simulink model "AIE_HDL"  (R2023a)
settings: Solver=FixedStepDiscrete  StartTime=0.0  StopTime=100*2e-9  RelTol=1e-3
InitFcn:
  | xlEvaluateHDLBlocks('AIE_HDL')
undefined symbols (not defined in the file): S, vsva2197, xcvc1902
libraries: hdlUtilities x4, dspsrcs4 x3, aieBasic x3, hdlBasic x2, vmcUtilities x1
settings Model: Creator=shirazi  LastModifiedBy=robg
settings SolverCC: AlgebraicLoopSolver=TrustRegion
settings DebuggingCC: UnconnectedInputMsg=warning  UnconnectedOutputMsg=warning  UnconnectedLineMsg=warning
settings ModelReferenceCC: EnableRefExpFcnMdlSchedulingChecks=on
settings SFSimCC: CustomCodeUndefinedFunction=UseInterfaceOnly
settings RTWCC: DLArmComputeVersion=19.05

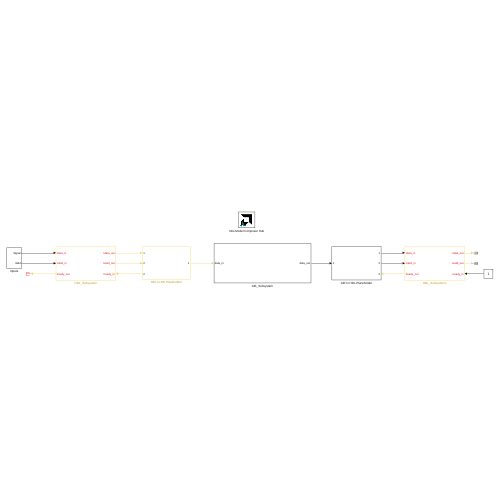
[thumbnail: Simulink's stored preview of the top-level diagram]
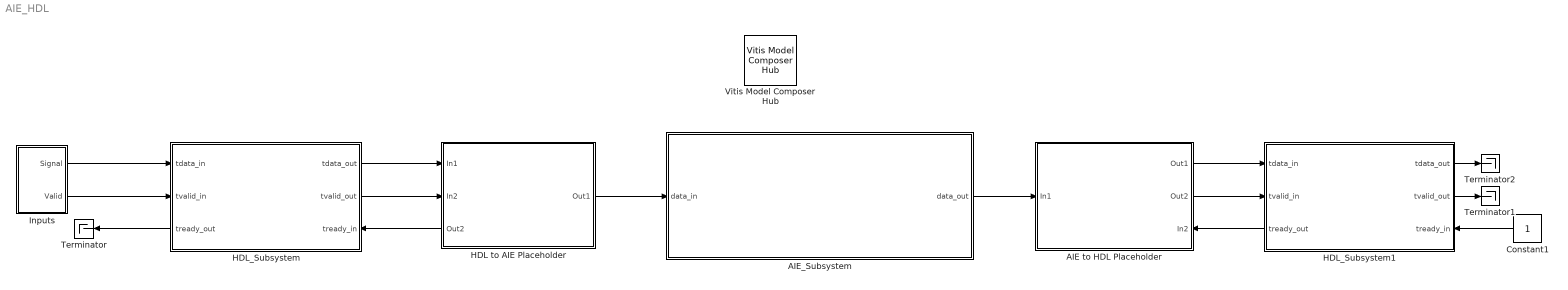
== system AIE_HDL ==
  AIE to HDL Placeholder : Subsystem
      settings: PortSchema="{\"entries\":[{\"content\":{\"sides\":[{\"content\":{\"connectorIds\":[\"In1\"]},\"type\":\"ConnectorPlacement.EquallySpacedRectSide\",\"uuid\":\"7ec462a4-9987-47a7-8ef6-3d77f6cbc297\"},{\"content\":{\"connectorIds\":[\"Out1\",\"Out2\",\"In2\"],\"side\":\"RIGHT\"},\"type\":\"ConnectorPlacement.EquallySpacedRectSide\",\"uuid\":\"048d0a02-5e23-4721-b2a0-067b0b8ade54\"},{\"content\":{\"connectorIds\":[],\"side\":\"TOP\"},\"type\":\"ConnectorPlacement.EquallySpacedRectSide\",\"uuid\":\"3a217202-6b4d-4910-945d-076f614a2b79\"}]},\"type\":\"ConnectorPlacement.EquallySpacedConnector\",\"uuid\":\"7ab6b02b-881c-4c80-a03f-a259c9ab4081\"}],\"packageUris\":[\"http://schema.mathworks.com/mf0/Connector/R2020b\"],\"version\":\"1.0\"}"
  AIE_Subsystem : Subsystem
  Constant1 : Constant  OutDataTypeStr=boolean  SampleTime=2e-9
  HDL to AIE Placeholder : Subsystem
      settings: PortSchema="{\"entries\":[{\"content\":{\"sides\":[{\"content\":{\"connectorIds\":[\"In1\",\"In2\",\"Out2\"]},\"type\":\"ConnectorPlacement.EquallySpacedRectSide\",\"uuid\":\"7ec462a4-9987-47a7-8ef6-3d77f6cbc297\"},{\"content\":{\"connectorIds\":[\"Out1\"],\"side\":\"RIGHT\"},\"type\":\"ConnectorPlacement.EquallySpacedRectSide\",\"uuid\":\"048d0a02-5e23-4721-b2a0-067b0b8ade54\"},{\"content\":{\"connectorIds\":[],\"side\":\"TOP\"},\"type\":\"ConnectorPlacement.EquallySpacedRectSide\",\"uuid\":\"3a217202-6b4d-4910-945d-076f614a2b79\"}]},\"type\":\"ConnectorPlacement.EquallySpacedConnector\",\"uuid\":\"7ab6b02b-881c-4c80-a03f-a259c9ab4081\"}],\"packageUris\":[\"http://schema.mathworks.com/mf0/Connector/R2020b\"],\"version\":\"1.0\"}"
  HDL_Subsystem : Subsystem
      settings: PortSchema="{\"entries\":[{\"content\":{\"sides\":[{\"content\":{\"connectorIds\":[\"In1\",\"In2\",\"Out3\"]},\"type\":\"ConnectorPlacement.EquallySpacedRectSide\",\"uuid\":\"989cb16a-31ef-4a7b-a4d3-adb9fa6297fb\"},{\"content\":{\"connectorIds\":[\"Out1\",\"Out2\",\"In3\"],\"side\":\"RIGHT\"},\"type\":\"ConnectorPlacement.EquallySpacedRectSide\",\"uuid\":\"9f541dfa-b9f2-4468-aad7-758d6944575e\"},{\"content\":{\"connectorIds\":[],\"side\":\"TOP\"},\"type\":\"ConnectorPlacement.EquallySpacedRectSide\",\"uuid\":\"c3c29352-583e-46d2-970b-15c15d07c124\"}]},\"type\":\"ConnectorPlacement.EquallySpacedConnector\",\"uuid\":\"c80158a0-6c2e-4236-83b1-850c61320738\"}],\"packageUris\":[\"http://schema.mathworks.com/mf0/Connector/19700101\"],\"version\":\"1.0\"}"
  HDL_Subsystem1 : Subsystem
      settings: PortSchema="{\"entries\":[{\"content\":{\"sides\":[{\"content\":{\"connectorIds\":[\"In1\",\"In2\",\"Out3\"]},\"type\":\"ConnectorPlacement.EquallySpacedRectSide\",\"uuid\":\"989cb16a-31ef-4a7b-a4d3-adb9fa6297fb\"},{\"content\":{\"connectorIds\":[\"Out1\",\"Out2\",\"In3\"],\"side\":\"RIGHT\"},\"type\":\"ConnectorPlacement.EquallySpacedRectSide\",\"uuid\":\"9f541dfa-b9f2-4468-aad7-758d6944575e\"},{\"content\":{\"connectorIds\":[],\"side\":\"TOP\"},\"type\":\"ConnectorPlacement.EquallySpacedRectSide\",\"uuid\":\"c3c29352-583e-46d2-970b-15c15d07c124\"}]},\"type\":\"ConnectorPlacement.EquallySpacedConnector\",\"uuid\":\"c80158a0-6c2e-4236-83b1-850c61320738\"}],\"packageUris\":[\"http://schema.mathworks.com/mf0/Connector/19700101\"],\"version\":\"1.0\"}"
  Inputs : Subsystem
  Terminator : Terminator
  Terminator1 : Terminator
  Terminator2 : Terminator
  Vitis Model Composer Hub : vmcUtilities/Vitis Model Composer Hub  Tag=genX  CodeGeneration=off  SubsystemName=HDL_Subsystem  StartColumn=1  NumberOfColumns=1  TargetDirectory=./code  exportDesign=off  analyzeDesign=off  validateDesignOnHw=off  ExportType=AI Engines  IpVendor=xilinx.com  IpLibrary=hls  IpVersion=1.0  IpHWLanguage=Verilog  AieCompilerOptions={}  AieSimulatorOptions={}  CreateTestbench=off  TestbenchStackSize=10  RunRtlSim=off  RunCSim=off  RunAieSim=off  AieSimTimeout=50000  RunAieSimProfiling=off  LaunchVitisAnalyzer=off  PlotOutput=off  RunX86Sim=off  X86SimTimeout=10  GenHwImage=off  GenLibadfXo=off  GenHwValidationCode=off  PlatformType=Not Specified  HwSystemType=Baremetal  HwValidationTarget=hw  ProjDevice=xcvc1902-vsva2197-1LP-e-S  ProjDevicePart=xcvc1902-vsva2197-1LP-e-S  AIEType=AIE  SamplePeriod=-1  ClockFrequency=200  DataPathParallelism=1  xilinxfamily=versalaicore  part=xcvc1902  speed=-1LP-e-S  package=vsva2197  directory=./netlist/ip/HDL_Subsystem/src  testbench=off  incr_netlist=off  synthesis_tool=Vivado  clock_wrapper=Clock Enables  dbl_ovrd=According to Block Masks  dcm_input_clock_period=10  sysclk_period=2  simulink_period=2e-9  eval_field=0  LogFileName=''  NThreads=4
  wires:
  HDL to AIE Placeholder/1(Out1) -> AIE_Subsystem/1(data_in)
  HDL_Subsystem/1(tdata_out) -> HDL to AIE Placeholder/1(In1)
  HDL_Subsystem/2(tvalid_out) -> HDL to AIE Placeholder/2(In2)
  HDL to AIE Placeholder/2(Out2) -> HDL_Subsystem/3(tready_in)
  HDL_Subsystem/3(tready_out) -> Terminator/1
  AIE_Subsystem/1(data_out) -> AIE to HDL Placeholder/1(In1)
  AIE to HDL Placeholder/1(Out1) -> HDL_Subsystem1/1(tdata_in)
  AIE to HDL Placeholder/2(Out2) -> HDL_Subsystem1/2(tvalid_in)
  HDL_Subsystem1/3(tready_out) -> AIE to HDL Placeholder/2(In2)
  Constant1/1 -> HDL_Subsystem1/3(tready_in)
  Inputs/1(Signal) -> HDL_Subsystem/1(tdata_in)
  Inputs/2(Valid) -> HDL_Subsystem/2(tvalid_in)
  HDL_Subsystem1/2(tvalid_out) -> Terminator1/1
  HDL_Subsystem1/1(tdata_out) -> Terminator2/1

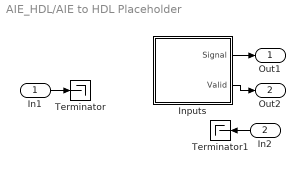
== system AIE_HDL/AIE to HDL Placeholder ==
  In1 : Inport
  In2 : Inport  Port=2
  Inputs : Subsystem
  Terminator : Terminator
  Terminator1 : Terminator
  Out1 : Outport
  Out2 : Outport  Port=2
  wires:
  Inputs/1(Signal) -> Out1/1
  Inputs/2(Valid) -> Out2/1
  In1/1 -> Terminator/1
  In2/1 -> Terminator1/1

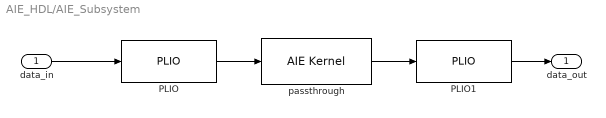
== system AIE_HDL/AIE_Subsystem ==
  data_in : Inport
  PLIO : aieBasic/PLIO  PlioWidth=64  PlioFreqSpec=on  PlioFreq=500  ColLocation=0  channel=0  blockJsonConstraints=[]  deprecateConstraints=0
  PLIO1 : aieBasic/PLIO  PlioWidth=64  PlioFreqSpec=on  PlioFreq=500  ColLocation=0  channel=0  blockJsonConstraints=[]  deprecateConstraints=0
  passthrough : aieBasic/AIE Kernel  KernelAllAttrs=|  PortNames={'in'; 'out'}  PortSerializedTypes={'{R{Tadf::input_buffer{1{t{Bi32}}}}}'; '{R{Tadf::output_buffer{1{t{Bi32}}}}}'}  PortWindowSizes={1.600000000000000000e+01, 1.600000000000000000e+01}  PortWindowMargins={0.000000000000000000e+00, 0.000000000000000000e+00}  PortSynchronicities={'sync', 'sync'}  PortSignalSizes={0.000000000000000000e+00; 0.000000000000000000e+00}  FunctionTemplateSpecKind=implicit  FunctionTemplateParamNames={'FRAME_LENGTH'}  FunctionTemplateParamKinds={'nontype'}  FunctionTemplateParamTypes={'int'}  FunctionTemplateParamValues={'16'}  FunctionIndex=1  FunctionTabVisible=on  FunctionTemplateParamsVisible=on  FunctionDeclTypeOptions=|  FunctionDecl=|  FunctionTemplateParams={ 'FRAME_LENGTH', 'int', '16' }  FunctionTemplateParamsEnables={'off', 'off', 'on'}  PortAttrs={ 'input', 'in', 'adf::input_buffer< int32 > &', '16', '0', 'sync', ''; 'output', 'out', 'adf::output_buffer< int32 > &', '16', '', 'sync', '' }  PortAttrsEnables={'off', 'off', 'off', 'on', 'off', 'off', 'off';'off', 'off', 'off', 'on', 'off', 'off', 'off'}  SampleTime=-1  KernelHeaderFile=passthrough.h  KernelFunction=passthrough  KernelSourceFile=passthrough.cc  KernelSearchPaths={}  PreProcOptions={}  blockJsonConstraints=[]
      KernelAllAttrs=|
      | s[12;12;9;9;19;14;21;23;21;23;24;21;15;17;12;24;26;26;26;27;28;9;21;23;23;23;24;25;14;19;19;29]@FunctionNameDeclFileNamePortNamesPortTypesPortSerializedTypesPortDirectionsPortWindowSizeEnablesPortWindowMarginEnablesPortBufferSizeEnablesPortBufferMarginEnablesPortSynchronicityEnablesPortSignalSizeEnablesPortBufferSizesPortBufferMarginsFunctionDeclFunctionTemplateSpecKindFunctionTemplateParamNamesFunctionTemplateParamKindsFunctionTemplateParamTypesFunctionTemplateParamValuesFunctionTemplateParamEnablesClassDeclClassTemplateSpecKindClassTemplateParamNamesClassTemplateParamKindsClassTemplateParamTypesClassTemplateParamValuesClassTemplateParamEnablesClassCtorDeclsClassCtorParamNamesClassCtorParamTypesClassCtorParamSerializedTypes[1 1]@C[32 1]@t11@passthrought19@../../passthrough.hC[2 1]@t2@int3@outC[2 1]@t28@adf::input_buffer< int32 > &t29@adf::output_buffer< int32 > &C[2 1]@t35@{R{Tadf::input_buffer{1{t{Bi32}}}}}t36@{R{Tadf::output_buffer{1{t{Bi32}}}}}C[2 1]@t5@inputt6@outputC[2 1]@l1@l1@C[2 1]@l1@l0@C[2 1]@l1@l1@C[2 1]@l0@l0@C[2 1]@l1@l1@C[2 1]@l0@l0@C[2 1]@nnC[2 1]@nnt115@template < int FRAME_LENGTH > 
      | void passthrough(adf::input_buffer< int32 > & in, adf::output_buffer< int32 > & out)t8@implicitC[1 1]@t12@FRAME_LENGTHC[1 1]@t7@nontypeC[1 1]@t3@intC[1 1]@nC[1 1]@l1@nne[0 1]@e[0 1]@e[0 1]@e[0 1]@e[0 1]@e[0 1]@e[0 1]@e[0 1]@e[0 1]@
      FunctionDeclTypeOptions=|
      | C[1 1]@t117@template < int FRAME_LENGTH > 
      | void passthrough(adf::input_buffer< int32 > && in, adf::output_buffer< int32 > && out)
      FunctionDecl=|
      | template < int FRAME_LENGTH > 
      | void passthrough(adf::input_buffer< int32 > && in, adf::output_buffer< int32 > && out)
  data_out : Outport
  wires:
  data_in/1 -> PLIO/1
  passthrough/1 -> PLIO1/1
  PLIO/1 -> passthrough/1
  PLIO1/1 -> data_out/1

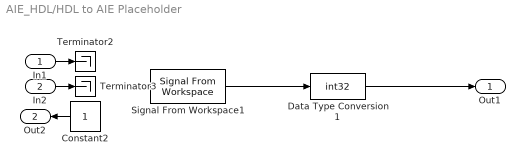
== system AIE_HDL/HDL to AIE Placeholder ==
  In1 : Inport
  In2 : Inport  Port=2
  Constant2 : Constant  OutDataTypeStr=boolean  SampleTime=2e-9
  Data Type Conversion1 : DataTypeConversion  OutDataTypeStr=int32  SaturateOnIntegerOverflow=off  RndMeth=Floor
  Signal From Workspace1 : dspsrcs4/Signal From Workspace  X=1:100  Ts=2e-9  nsamps=16  OutputAfterFinalValue=Cyclic repetition  ignoreOrWarnInputAndFrameLengths=off  OutputFrames=off
  Terminator2 : Terminator
  Terminator3 : Terminator
  Out1 : Outport
  Out2 : Outport  Port=2
  wires:
  Signal From Workspace1/1 -> Data Type Conversion1/1
  Constant2/1 -> Out2/1
  In1/1 -> Terminator2/1
  In2/1 -> Terminator3/1
  Data Type Conversion1/1 -> Out1/1

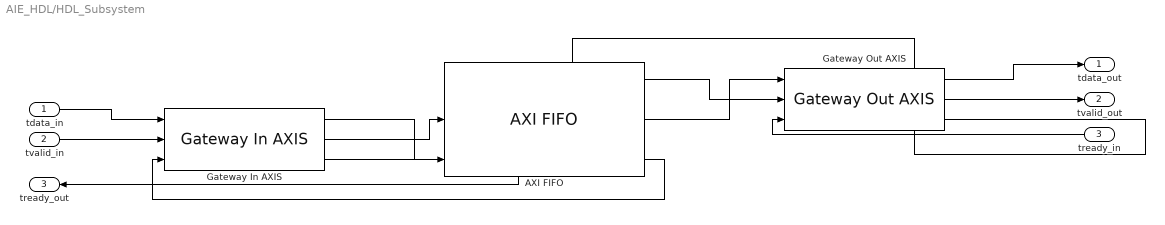
== system AIE_HDL/HDL_Subsystem ==
  tdata_in : Inport
  tvalid_in : Inport  Port=2
  tready_in : Inport  Port=3
  AXI FIFO : hdlBasic/AXI FIFO  input_depth_axis=16  actual_fifo_depth_label=18  enable_tdata=on  enable_tdest=off  enable_tstrb=off  enable_tready=on  enable_tid=off  enable_tuser=off  enable_tkeep=off  enable_tlast=off  has_aresetn=off  enable_data_counts_axis=off  fifo_implementation_type_axis=Common Clock Block RAM  trim_axipin_name=off  programmable_full_type_axis=Full  full_threshold_assert_value_axis=0  programmable_empty_type_axis=Empty  empty_threshold_assert_value_axis=1022  underflow_flag_axi=0  underflow_sense_axi=Active High  overflow_flag_axi=0  overflow_sense_axi=Active High  simulation_type=fast_sim  XmcBlockStatus=1  maskContainerNames=tabcontainer1  block_type=axi_fifo  block_config=sysgen:AXI_FIFO_config
  Gateway In AXIS : hdlUtilities/Gateway In AXIS  gui_display_data_type=Fixed-point  arith_type=Unsigned  n_bits=64  bin_pt=0  preci_type=Custom  exp_width=16  frac_width=24  quantization=Truncate  overflow=Flag as error  OutSampleTime=2e-9  block_type=gatewayinaxi  XmcBlockStatus=1
      link override Gateway In AXIS_tdata: arith_type=Unsigned
  Gateway Out AXIS : hdlUtilities/Gateway Out AXIS  mask_sample_period=2e-9  block_type=gatewayoutaxi
  tdata_out : Outport
  tvalid_out : Outport  Port=2
  tready_out : Outport  Port=3
  wires:
  AXI FIFO/2 -> Gateway Out AXIS/1
  AXI FIFO/1 -> Gateway Out AXIS/2
  tready_in/1 -> Gateway Out AXIS/3
  AXI FIFO/3 -> Gateway In AXIS/3
  tvalid_in/1 -> Gateway In AXIS/2
  tdata_in/1 -> Gateway In AXIS/1
  Gateway Out AXIS/3 -> AXI FIFO/1
  Gateway In AXIS/3 -> tready_out/1
  Gateway Out AXIS/2 -> tvalid_out/1
  Gateway Out AXIS/1 -> tdata_out/1
  Gateway In AXIS/1 -> AXI FIFO/3
  Gateway In AXIS/2 -> AXI FIFO/2

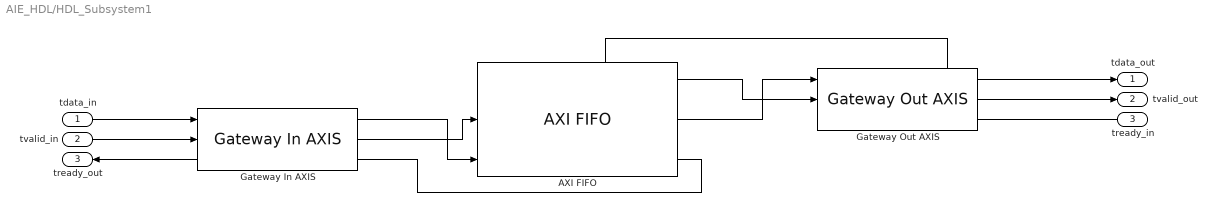
== system AIE_HDL/HDL_Subsystem1 ==
  tdata_in : Inport
  tvalid_in : Inport  Port=2
  tready_in : Inport  Port=3
  AXI FIFO : hdlBasic/AXI FIFO  input_depth_axis=1K  actual_fifo_depth_label=1026  enable_tdata=on  enable_tdest=off  enable_tstrb=off  enable_tready=on  enable_tid=off  enable_tuser=off  enable_tkeep=off  enable_tlast=off  has_aresetn=off  enable_data_counts_axis=off  fifo_implementation_type_axis=Common Clock Block RAM  trim_axipin_name=off  programmable_full_type_axis=Full  full_threshold_assert_value_axis=0  programmable_empty_type_axis=Empty  empty_threshold_assert_value_axis=1022  underflow_flag_axi=0  underflow_sense_axi=Active High  overflow_flag_axi=0  overflow_sense_axi=Active High  simulation_type=fast_sim  XmcBlockStatus=1  maskContainerNames=tabcontainer1  block_type=axi_fifo  block_config=sysgen:AXI_FIFO_config
  Gateway In AXIS : hdlUtilities/Gateway In AXIS  gui_display_data_type=Fixed-point  arith_type=Unsigned  n_bits=64  bin_pt=0  preci_type=Custom  exp_width=16  frac_width=24  quantization=Truncate  overflow=Flag as error  OutSampleTime=2e-9  block_type=gatewayinaxi  XmcBlockStatus=1
      link override Gateway In AXIS_tdata: arith_type=Unsigned
  Gateway Out AXIS : hdlUtilities/Gateway Out AXIS  mask_sample_period=2e-9  block_type=gatewayoutaxi
  tdata_out : Outport
  tvalid_out : Outport  Port=2
  tready_out : Outport  Port=3
  wires:
  AXI FIFO/2 -> Gateway Out AXIS/1
  AXI FIFO/1 -> Gateway Out AXIS/2
  tready_in/1 -> Gateway Out AXIS/3
  AXI FIFO/3 -> Gateway In AXIS/3
  tvalid_in/1 -> Gateway In AXIS/2
  tdata_in/1 -> Gateway In AXIS/1
  Gateway Out AXIS/3 -> AXI FIFO/1
  Gateway In AXIS/3 -> tready_out/1
  Gateway Out AXIS/2 -> tvalid_out/1
  Gateway Out AXIS/1 -> tdata_out/1
  Gateway In AXIS/1 -> AXI FIFO/3
  Gateway In AXIS/2 -> AXI FIFO/2

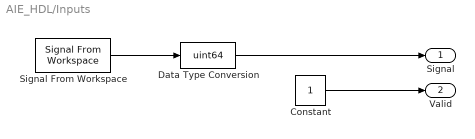
== system AIE_HDL/Inputs ==
  Constant : Constant  OutDataTypeStr=boolean  SampleTime=2e-9
  Data Type Conversion : DataTypeConversion  OutDataTypeStr=uint64  SaturateOnIntegerOverflow=off  RndMeth=Floor
  Signal From Workspace : dspsrcs4/Signal From Workspace  X=1:100  Ts=2e-9  nsamps=1  OutputAfterFinalValue=Cyclic repetition  ignoreOrWarnInputAndFrameLengths=off  OutputFrames=off
  Signal : Outport
  Valid : Outport  Port=2
  wires:
  Data Type Conversion/1 -> Signal/1
  Constant/1 -> Valid/1
  Signal From Workspace/1 -> Data Type Conversion/1

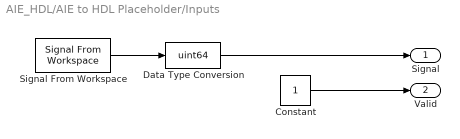
== system AIE_HDL/AIE to HDL Placeholder/Inputs ==
  Constant : Constant  OutDataTypeStr=boolean  SampleTime=2e-9
  Data Type Conversion : DataTypeConversion  OutDataTypeStr=uint64  SaturateOnIntegerOverflow=off  RndMeth=Floor
  Signal From Workspace : dspsrcs4/Signal From Workspace  X=1:100  Ts=2e-9  nsamps=1  OutputAfterFinalValue=Cyclic repetition  ignoreOrWarnInputAndFrameLengths=off  OutputFrames=off
  Signal : Outport
  Valid : Outport  Port=2
  wires:
  Signal From Workspace/1 -> Data Type Conversion/1
  Data Type Conversion/1 -> Signal/1
  Constant/1 -> Valid/1
